simulink library "Lib_PFSys_BiDirGenericMotor_TMATS"  (R2017a)
settings: Solver=ode45  StartTime=0.0  StopTime=10.0  RelTol=1e-3  EnableMultiTasking=on
libraries: Lib_PF_BusLoadDC_TMATS x1, Lib_PF_LineDC_TMATS x1
Description:
  | Thomas Modules
settings Model: Creator=jwchapm2  LastModifiedBy=glthoma1
settings DataIOCC: LimitDataPoints=on  SaveFormat=Array
settings OptimizationCC: ExpressionDepthLimit=2147483647  LifeSpan=inf
settings DebuggingCC: UnderspecifiedInitializationDetection=Classic  MergeDetectMultiDrivingBlocksExec=none  SolverPrmCheckMsg=warning  StateNameClashWarn=warning  SFUnexpectedBacktrackingDiag=warning  SFNoUnconditionalDefaultTransitionDiag=warning  SFExecutionAtInitializationDiag=none
settings HardwareCC: ProdBitPerPointer=32  ProdBitPerSizeT=32  ProdBitPerPtrDiffT=32  ProdLargestAtomicFloat=None  ProdIntDivRoundTo=Undefined  ProdEndianess=Unspecified  ProdWordSize=32  ProdHWDeviceType=32-bit Generic
settings ModelReferenceCC: PropagateSignalLabelsOutOfModel=off
settings GRTTargetCC: TargetLangStandard=C89/C90 (ANSI)  GeneratePreprocessorConditionals=Disable all
settings ConfigComp: CovMetricSettings=dw  CovHtmlReporting=on  CovSaveCumulativeToWorkspaceVar=on  CovSaveSingleToWorkspaceVar=on  CovExternalEMLEnable=off

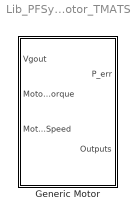
== system Lib_PFSys_BiDirGenericMotor_TMATS ==
  Generic Motor : Subsystem  mask(Motor){X_C_TorqueVec_M=[0 1000 10000], Y_C_SpeedVec_M=[0 500 5000], T_C_EffArray_M=[0.5 0.5 0.5; 0.5 1 1; 0.5 1 1], Z_M=0.01}
      mask prompts: X_C_TorqueVec_M "X_C_TorqueVec_M - Efficiency Table Torque Vector (X-axis)(nx1)"; Y_C_SpeedVec_M "Y_C_SpeedVec_M - Efficiency Table Speed Vector (Y-axis)(mx1)"; T_C_EffArray_M "T_C_EffArray_M - Efficiency Table Values (Eff = f(i, V)(nxm)"; Z_M "Z_M - Resistive Impedance"
      mask help: This block represents a generic motor with a standard resistive impedance of 0.01 Ohms and an efficiency table input.

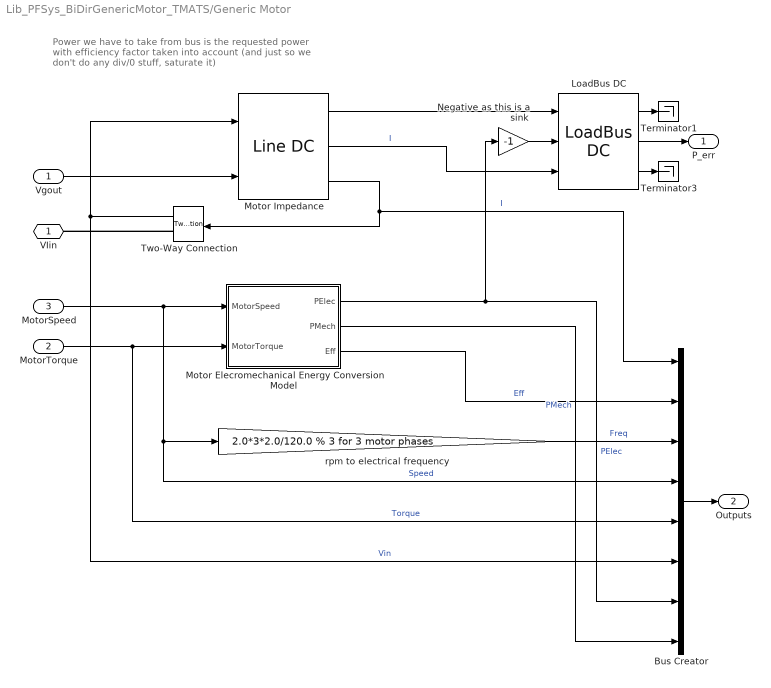
== system Lib_PFSys_BiDirGenericMotor_TMATS/Generic Motor ==
  note: Power we have to take from bus is the requested power
      | with efficiency factor taken into account
      | (and just so we don't do any div/0 stuff, saturate it)
  Vgout : Inport
  MotorTorque : Inport  Port=2
  MotorSpeed : Inport  Port=3
  Bus Creator : BusCreator  Inputs=8
  LoadBus DC : Lib_PF_BusLoadDC_TMATS/LoadBus DC  PeInEN_M=on  P_M=-2  BlkNm_M=double(gcb)
  Motor Elecromechanical Energy Conversion Model : Subsystem
  Motor Impedance : Lib_PF_LineDC_TMATS/Line DC  R_M=Z_M
  Negative as this is a sink : Gain  Gain=-1
  Terminator1 : Terminator
  Terminator3 : Terminator
  Two-Way Connection : TwoWayConnection
  rpm to electrical frequency : Gain  Gain=2.0*3*2.0/120.0 % 3 for 3 motor phases
  VIin : PMIOPort  Port=1  Side=Left
  P_err : Outport
  Outputs : Outport  Port=2
  wires:
  Negative as this is a sink/1 -> LoadBus DC/2
  Motor Impedance/2 -> LoadBus DC/3  "I"
  Motor Impedance/3 -> Bus Creator/1, Two-Way Connection/1  "I"
  Motor Impedance/1 -> LoadBus DC/1
  Vgout/1 -> Motor Impedance/2
  Bus Creator/1 -> Outputs/1
  rpm to electrical frequency/1 -> Bus Creator/3  "Freq"
  MotorTorque/1 -> Bus Creator/5, Motor Elecromechanical Energy Conversion Model/2(MotorTorque)  "Torque"
  MotorSpeed/1 -> rpm to electrical frequency/1, Bus Creator/4, Motor Elecromechanical Energy Conversion Model/1(MotorSpeed)  "Speed"
  LoadBus DC/3 -> Terminator3/1
  Two-Way Connection/1 -> Motor Impedance/1, Bus Creator/6  "Vin"
  LoadBus DC/2 -> P_err/1
  LoadBus DC/1 -> Terminator1/1
  Motor Elecromechanical Energy Conversion Model/1(PElec) -> Negative as this is a sink/1, Bus Creator/7  "PElec"
  Motor Elecromechanical Energy Conversion Model/3(Eff) -> Bus Creator/2  "Eff"
  Motor Elecromechanical Energy Conversion Model/2(PMech) -> Bus Creator/8  "PMech"
  connections:
  Two-Way Connection/RConn1 -- VIin/RConn1

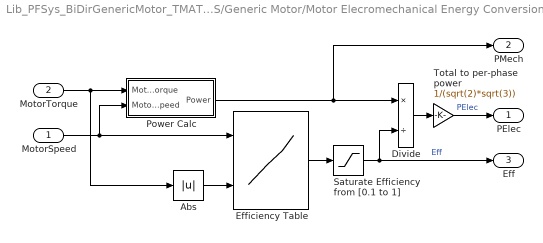
== system Lib_PFSys_BiDirGenericMotor_TMATS/Generic Motor/Motor Elecromechanical Energy Conversion Model ==
  MotorSpeed : Inport
  MotorTorque : Inport  Port=2
  Abs : Abs
  Divide : Product  Inputs=*/
  Efficiency Table : Lookup_n-D  BreakpointsForDimension1=X_C_TorqueVec_M  BreakpointsForDimension2=Y_C_SpeedVec_M  Table=T_C_EffArray_M  ExtrapMethod=Clip  InternalRulePriority=Speed  RndMeth=Simplest  InputSameDT=on
  Power Calc : Subsystem
  Saturate Efficiency from [0.1 to 1] : Saturate  UpperLimit=1  LowerLimit=0.1
  Total to per-phase power : Gain  Gain=1/(sqrt(2)*sqrt(3))
  PElec : Outport
  PMech : Outport  Port=2
  Eff : Outport  Port=3
  wires:
  Efficiency Table/1 -> Saturate Efficiency from [0.1 to 1]/1
  Saturate Efficiency from [0.1 to 1]/1 -> Eff/1, Divide/2  "Eff"
  Abs/1 -> Efficiency Table/2
  Total to per-phase power/1 -> PElec/1  "PElec"
  Divide/1 -> Total to per-phase power/1
  Power Calc/1(Power) -> PMech/1, Divide/1
  MotorTorque/1 -> Abs/1, Power Calc/1(MotorTorque)
  MotorSpeed/1 -> Power Calc/2(MotorSpeed), Efficiency Table/1

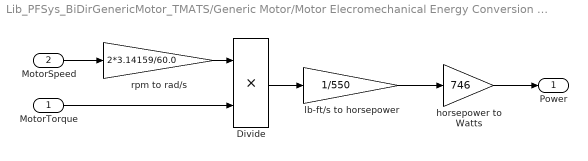
== system Lib_PFSys_BiDirGenericMotor_TMATS/Generic Motor/Motor Elecromechanical Energy Conversion Model/Power Calc ==
  MotorTorque : Inport
  MotorSpeed : Inport  Port=2
  Divide : Product  Inputs=**
  horsepower to Watts : Gain  Gain=746
  lb-ft/s to horsepower : Gain  Gain=1/550
  rpm to rad/s : Gain  Gain=2*3.14159/60.0
  Power : Outport
  wires:
  MotorSpeed/1 -> rpm to rad/s/1
  Divide/1 -> lb-ft/s to horsepower/1
  lb-ft/s to horsepower/1 -> horsepower to Watts/1
  MotorTorque/1 -> Divide/2
  rpm to rad/s/1 -> Divide/1
  horsepower to Watts/1 -> Power/1
